simulink model "Centralized_Control_G18"  (R2020a)
settings: Solver=VariableStepAuto  StartTime=0.0  StopTime=60  RelTol=1e-3
values from neighbouring files (symbols this model uses):
  CK_dH = CK_dL.*5    [Dynamics_G18.m]
  CK_dL = diag([40; 40; 40; 40; 40; 40])    [Dynamics_G18.m]
  CK_dM = CK_dL.*3    [Dynamics_G18.m]
  CK_pH = CK_pL.*25    [Dynamics_G18.m]
  CK_pL = diag([400; 400; 400; 400; 400; 400])    [Dynamics_G18.m]
  CK_pM = CK_pL.*9    [Dynamics_G18.m]
  DH = [ 0.089    q1     0    pi/2    0     'R' ... (first row only)    [Robot_G18.m]
libraries: vrlib x7, dspinverses x2, aerolibanimutils x1, RobotG18_Blocos x1, simulink x1
settings Model: Creator=Ricardo Henriques  LastModifiedBy=Catarina
settings DataIOCC: ReturnWorkspaceOutputs=off
settings OptimizationCC: LifeSpan=inf
settings DebuggingCC: ArithmeticOperatorsInVariantConditions=warning
settings SFSimCC: SimUseLocalCustomCode=off  CustomCodeUndefinedFunction=UseInterfaceOnly
settings RTWCC: RTWUseLocalCustomCode=off
settings CodeAppCC: StateflowObjectComments=on

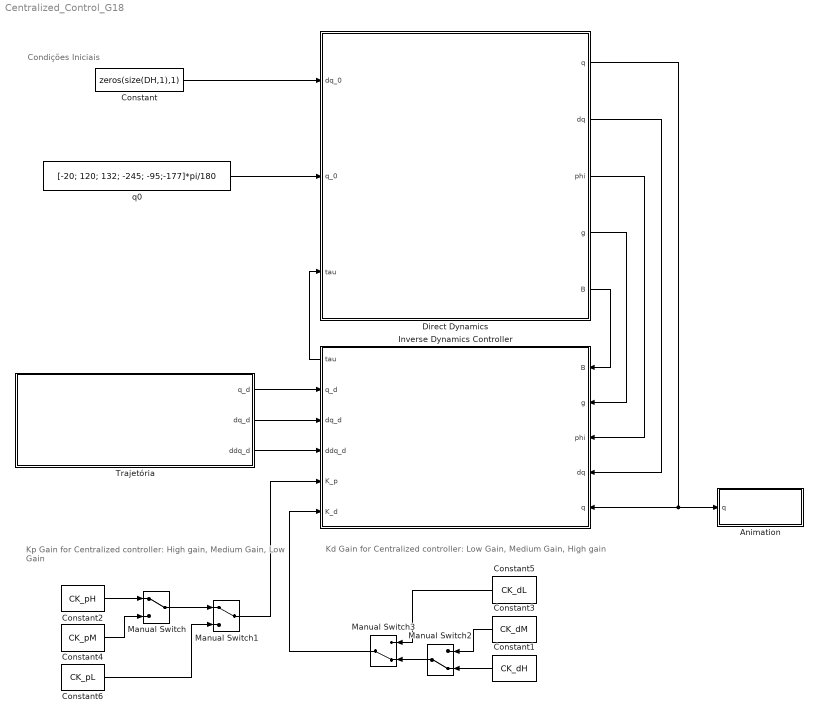
== system Centralized_Control_G18 ==
  note: Kd Gain for Centralized controller:
      |  Low Gain, Medium Gain, High gain
  note: Kp Gain for Centralized controller:
      | High gain, Medium Gain, Low Gain
  note: Condições Iniciais
  "Animation " : Subsystem
  Constant : Constant  Value=zeros(size(DH,1),1)  VectorParams1D=off
  Constant1 : Constant  Value=CK_dH  VectorParams1D=off
  Constant2 : Constant  Value=CK_pH  VectorParams1D=off
  Constant3 : Constant  Value=CK_dM  VectorParams1D=off
  Constant4 : Constant  Value=CK_pM  VectorParams1D=off
  Constant5 : Constant  Value=CK_dL  VectorParams1D=off
  Constant6 : Constant  Value=CK_pL  VectorParams1D=off
  Direct Dynamics : Subsystem
  Inverse Dynamics Controller : Subsystem
      settings: PortSchema="{\"entries\":[{\"content\":{\"sides\":[{\"content\":{\"connectorIds\":[\"In1\",\"In2\",\"In3\",\"In4\",\"In5\"]},\"type\":\"ConnectorPlacement.EquallySpacedRectSide\",\"uuid\":\"0e680a2d-49f3-406c-b827-b0951d4aa640\"},{\"content\":{\"connectorIds\":[\"Out1\",\"In6\",\"In7\",\"In8\",\"In9\",\"In10\"],\"side\":\"RIGHT\"},\"type\":\"ConnectorPlacement.EquallySpacedRectSide\",\"uuid\":\"bf9b0e73-475c-43b8-a2d1-242f88155fc5\"},{\"content\":{\"connectorIds\":[],\"side\":\"TOP\"},\"type\":\"ConnectorPlacement.EquallySpacedRectSide\",\"uuid\":\"dd2b5620-6d82-4ff2-af29-930996194164\"}]},\"type\":\"ConnectorPlacement.EquallySpacedConnector\",\"uuid\":\"c87e6944-d8f4-4feb-bccd-937ad879e06a\"}],\"packageUris\":[\"http://schema.mathworks.com/mf0/Connector/19700101\"],\"version\":\"1.0\"}"
  Manual Switch : ManualSwitch
  Manual Switch1 : ManualSwitch
  Manual Switch2 : ManualSwitch  CurrentSetting=0
  Manual Switch3 : ManualSwitch  CurrentSetting=0
  Trajetória : Subsystem
  q0 : Constant  Value=[-20; 120; 132; -245; -95;-177]*pi/180  VectorParams1D=off
  wires:
  Constant/1 -> Direct Dynamics/1(dq_0)
  Direct Dynamics/5(B) -> Inverse Dynamics Controller/1(B)
  Direct Dynamics/4(g) -> Inverse Dynamics Controller/2(g)
  Direct Dynamics/3(phi) -> Inverse Dynamics Controller/3(phi)
  Direct Dynamics/2(dq) -> Inverse Dynamics Controller/4(dq)
  Direct Dynamics/1(q) -> "Animation "/1("q "), Inverse Dynamics Controller/5(q)
  Inverse Dynamics Controller/1(tau) -> Direct Dynamics/3(tau)
  q0/1 -> Direct Dynamics/2(q_0)
  Trajetória/3(ddq_d) -> Inverse Dynamics Controller/8(ddq_d)
  Constant2/1 -> Manual Switch/1
  Constant4/1 -> Manual Switch/2
  Manual Switch/1 -> Manual Switch1/1
  Manual Switch1/1 -> Inverse Dynamics Controller/9(K_p)
  Constant6/1 -> Manual Switch1/2
  Constant1/1 -> Manual Switch2/2
  Constant3/1 -> Manual Switch2/1
  Manual Switch2/1 -> Manual Switch3/2
  Manual Switch3/1 -> Inverse Dynamics Controller/10(K_d)
  Constant5/1 -> Manual Switch3/1
  Trajetória/2(dq_d) -> Inverse Dynamics Controller/7(dq_d)
  Trajetória/1(q_d) -> Inverse Dynamics Controller/6(q_d)

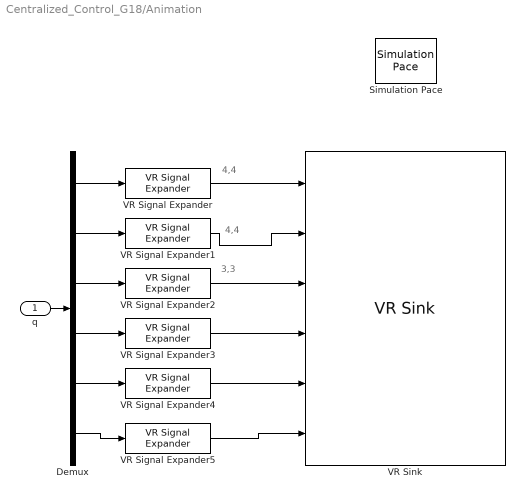
== system Centralized_Control_G18/Animation  ==
  note: 4,4
  note: 3,3
  note: 4,4
  "q " : Inport
  Demux : Demux  Outputs=6
  Simulation Pace : aerolibanimutils/Simulation Pace  SimulationPace=1  SleepMode=Auto  OutputPaceError=off  SampleTime=1/30
  VR Signal Expander{,1..5} (6 alike) : vrlib/VR Signal Expander  outwidth=4  outidx=4
  VR Sink : vrlib/VR Sink  InstantiateOnLoad=on  SampleTime=1/30  ViewEnable=on  RemoteChange=off  RemoteView=off  FieldsWritten=Jt1_DH_dv.rotation.4.1.1.double#Jt2_DH_dv.rotation.4.1.1.double#Jt3_DH_dv.rotation.4.1.1.double#Jt4_DH_dv.rotation.4.1.1.double#Jt5_DH_dv.rotation.4.1.1.double#Jt6_DH_dv.rotation.4.1.1.double  WorldFileName=RobotG18_Opt_NoAxes.wrl  WorldDescription=D-H Reference Frames for Virtual Reality Robot  AutoView=off  VideoDimensions=[]  AllowVariableSize=off
  wires:
  "q "/1 -> Demux/1
  Demux/1 -> VR Signal Expander/1
  Demux/2 -> VR Signal Expander1/1
  Demux/3 -> VR Signal Expander2/1
  Demux/4 -> VR Signal Expander3/1
  Demux/5 -> VR Signal Expander4/1
  Demux/6 -> VR Signal Expander5/1
  VR Signal Expander/1 -> VR Sink/1
  VR Signal Expander1/1 -> VR Sink/2
  VR Signal Expander5/1 -> VR Sink/6
  VR Signal Expander2/1 -> VR Sink/3
  VR Signal Expander3/1 -> VR Sink/4
  VR Signal Expander4/1 -> VR Sink/5

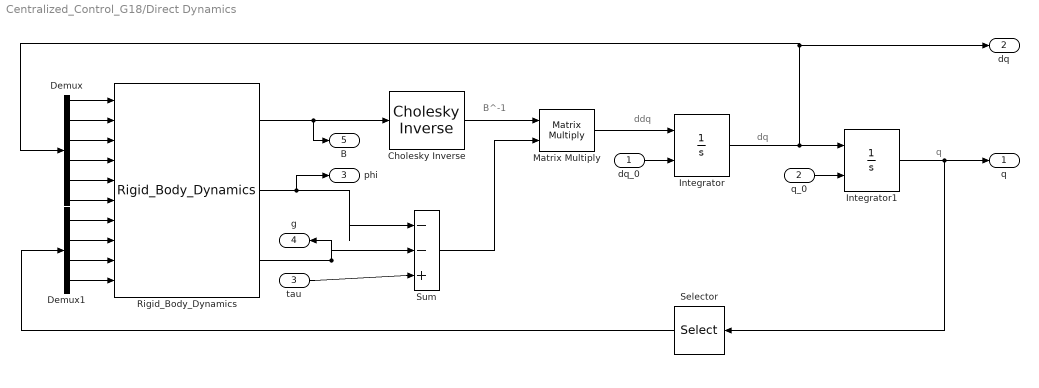
== system Centralized_Control_G18/Direct Dynamics ==
  note: q
  note: dq
  note: ddq
  note: B^-1
  dq_0 : Inport
  q_0 : Inport  Port=2
  tau : Inport  Port=3
  Cholesky Inverse : dspinverses/Cholesky Inverse  errmode=Warning
      settings: SourceProductBaseCode=DS
  Demux : Demux  Outputs=6
  Demux1 : Demux
  Integrator : Integrator  InitialConditionSource=external
  Integrator1 : Integrator  InitialConditionSource=external
  Matrix Multiply : Product  Multiplication=Matrix(*)
  Rigid_Body_Dynamics : RobotG18_Blocos/Rigid_Body_Dynamics  SystemSampleTime=-1  Latency=0  AutoFrameSizeCalculation=off
  Selector : Selector  InputPortWidth=6  IndexOptions=Index vector (dialog)  Indices=[2 3 4 5]  OutputSizes=1
  Sum : Sum  Inputs=|--+
  q : Outport
  dq : Outport  Port=2
  phi : Outport  Port=3
  g : Outport  Port=4
  B : Outport  Port=5
  wires:
  dq_0/1 -> Integrator/2
  Integrator1/1 -> q/1, Selector/1
  q_0/1 -> Integrator1/2
  Matrix Multiply/1 -> Integrator/1
  Cholesky Inverse/1 -> Matrix Multiply/1
  Sum/1 -> Matrix Multiply/2
  Rigid_Body_Dynamics/1 -> B/1, Cholesky Inverse/1
  tau/1 -> Sum/3
  Rigid_Body_Dynamics/3 -> g/1, Sum/2
  Rigid_Body_Dynamics/2 -> phi/1, Sum/1
  Demux/1 -> Rigid_Body_Dynamics/1
  Demux/2 -> Rigid_Body_Dynamics/2
  Demux/3 -> Rigid_Body_Dynamics/3
  Demux/4 -> Rigid_Body_Dynamics/4
  Demux/5 -> Rigid_Body_Dynamics/5
  Demux/6 -> Rigid_Body_Dynamics/6
  Demux1/1 -> Rigid_Body_Dynamics/7
  Demux1/2 -> Rigid_Body_Dynamics/8
  Demux1/3 -> Rigid_Body_Dynamics/9
  Demux1/4 -> Rigid_Body_Dynamics/10
  Selector/1 -> Demux1/1
  Integrator/1 -> Demux/1, dq/1, Integrator1/1

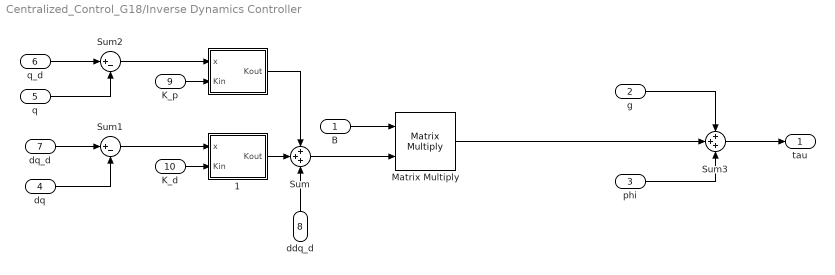
== system Centralized_Control_G18/Inverse Dynamics Controller ==
  B : Inport
  g : Inport  Port=2
  phi : Inport  Port=3
  dq : Inport  Port=4
  q : Inport  Port=5
  q_d : Inport  Port=6
  dq_d : Inport  Port=7
  ddq_d : Inport  Port=8
  K_p : Inport  Port=9
  K_d : Inport  Port=10
  " " : MATLAB Function  TreatAsAtomicUnit=on
  " 1" : MATLAB Function  TreatAsAtomicUnit=on
  Matrix Multiply : Product  Multiplication=Matrix(*)
  Sum : Sum  Inputs=+++
  Sum1 : Sum  Inputs=|+-
  Sum2 : Sum  Inputs=|+-
  Sum3 : Sum  Inputs=+++
  tau : Outport
  wires:
  Sum1/1 -> " 1"/1(x)
  Sum/1 -> Matrix Multiply/2
  ddq_d/1 -> Sum/3
  " 1"/1(Kout) -> Sum/2
  dq_d/1 -> Sum1/1
  Sum2/1 -> " "/1(x)
  q_d/1 -> Sum2/1
  Sum3/1 -> tau/1
  g/1 -> Sum3/1
  B/1 -> Matrix Multiply/1
  phi/1 -> Sum3/3
  Matrix Multiply/1 -> Sum3/2
  q/1 -> Sum2/2
  dq/1 -> Sum1/2
  " "/1(Kout) -> Sum/1
  K_p/1 -> " "/2(Kin)
  K_d/1 -> " 1"/2(Kin)

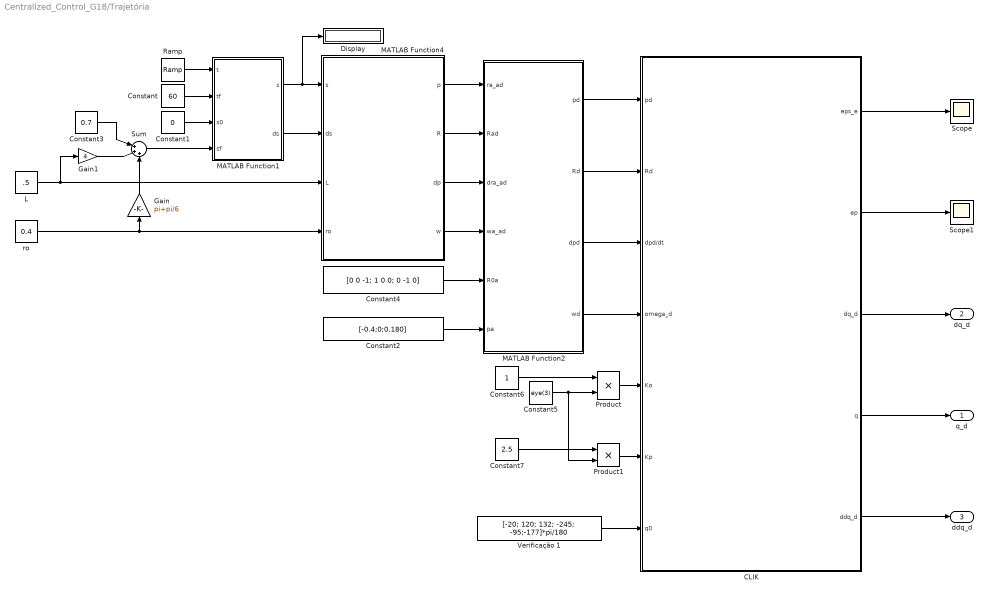
== system Centralized_Control_G18/Trajetória ==
  CLIK : Subsystem
  Constant : Constant  Value=60
  Constant1 : Constant  Value=0
  Constant2 : Constant  Value=[-0.4;0;0.180]  VectorParams1D=off
  Constant3 : Constant  Value=0.7
  Constant4 : Constant  Value=[0 0 -1; 1 0 0; 0 -1 0]  VectorParams1D=off
  Constant5 : Constant  Value=eye(3)
  Constant6 : Constant
  Constant7 : Constant  Value=2.5
  Display : Display
  Gain : Gain  Gain=pi+pi/6
  Gain1 : Gain  Gain=4
  L : Constant  Value=.5
  MATLAB Function1 : MATLAB Function  TreatAsAtomicUnit=on
  MATLAB Function2 : MATLAB Function  TreatAsAtomicUnit=on
  MATLAB Function4 : MATLAB Function  TreatAsAtomicUnit=on
  Product : Product
  Product1 : Product
  Ramp : simulink/Sources/Ramp  slope=1  start=0  InitialOutput=0
  Scope : Scope
  Scope1 : Scope
  Sum : Sum  Inputs=|+++
  Verificação 1 : Constant  Value=[-20; 120; 132; -245; -95;-177]*pi/180  VectorParams1D=off  SampleTime=inf
  ro : Constant  Value=0.4
  q_d : Outport
  dq_d : Outport  Port=2
  ddq_d : Outport  Port=3
  wires:
  MATLAB Function2/2(Rd) -> CLIK/2(Rd)
  Product1/1 -> CLIK/6(Kp)
  Constant4/1 -> MATLAB Function2/5(R0a)
  Gain/1 -> Sum/3
  CLIK/3(dq_d) -> dq_d/1
  CLIK/2(ep) -> Scope1/1
  CLIK/4(q) -> q_d/1
  Constant/1 -> MATLAB Function1/2(tf)
  Constant1/1 -> MATLAB Function1/3(s0)
  CLIK/1(eps_e) -> Scope/1
  Constant3/1 -> Sum/1
  Constant7/1 -> Product1/1
  MATLAB Function4/4(w) -> MATLAB Function2/4(wa_ad)
  Constant6/1 -> Product/1
  MATLAB Function1/2(ds) -> MATLAB Function4/2(ds)
  MATLAB Function2/3(dpd) -> CLIK/3(dpd/dt)
  Verificação 1/1 -> CLIK/7(q0)
  Sum/1 -> MATLAB Function1/4(sf)
  ro/1 -> MATLAB Function4/4(ro), Gain/1
  MATLAB Function4/3(dp) -> MATLAB Function2/3(dra_ad)
  MATLAB Function2/1(pd) -> CLIK/1(pd)
  Ramp/1 -> MATLAB Function1/1(t)
  Constant5/1 -> Product1/2, Product/2
  Constant2/1 -> MATLAB Function2/6(pa)
  MATLAB Function2/4(wd) -> CLIK/4(omega_d)
  Product/1 -> CLIK/5(Ko)
  MATLAB Function4/1(p) -> MATLAB Function2/1(ra_ad)
  Gain1/1 -> Sum/2
  MATLAB Function1/1(s) -> MATLAB Function4/1(s), Display/1
  MATLAB Function4/2(R) -> MATLAB Function2/2(Rad)
  L/1 -> MATLAB Function4/3(L), Gain1/1
  CLIK/5(ddq_d) -> ddq_d/1

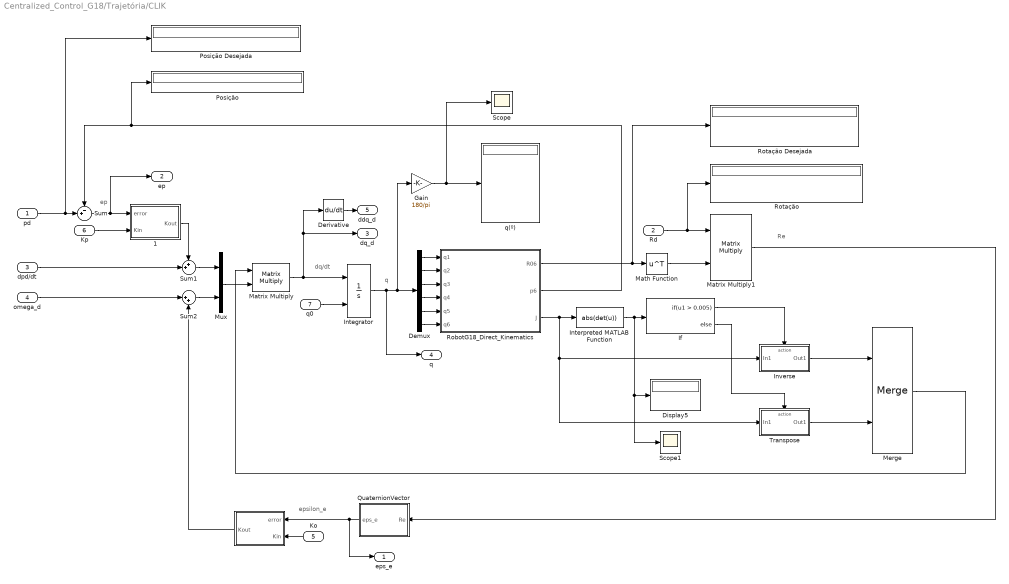
== system Centralized_Control_G18/Trajetória/CLIK ==
  note: epsilon_e
  note: Re
  note: ep
  note: dq/dt
  note: q
  pd : Inport
  Rd : Inport  Port=2
  dpd/dt : Inport  Port=3
  omega_d : Inport  Port=4
  Ko : Inport  Port=5
  Kp : Inport  Port=6
  q0 : Inport  Port=7
  " " : MATLAB Function  TreatAsAtomicUnit=on
  " 1" : MATLAB Function  TreatAsAtomicUnit=on
  Demux : Demux  Outputs=6
  Derivative : Derivative
  Display5 : Display
  Gain : Gain  Gain=180/pi
  If : If  IfExpression=u1 > 0.005  ZeroCross=off
  Integrator : Integrator  InitialConditionSource=external
  Interpreted MATLAB Function : MATLABFcn  MATLABFcn=abs(det(u))
  Inverse : Subsystem  TreatAsAtomicUnit=on
  Math Function : Math  Operator=transpose  SignedPower=on  SaturateOnIntegerOverflow=on
  Matrix Multiply : Product  Multiplication=Matrix(*)
  Matrix Multiply1 : Product  Multiplication=Matrix(*)
  Merge : Merge
  Mux : Mux  Inputs=2
  Posição : Display
      settings: Decimation=3
  Posição Desejada : Display
      settings: Decimation=3
  QuaternionVector : MATLAB Function  TreatAsAtomicUnit=on
  RobotG18_Direct_Kinematics : MATLAB Function  TreatAsAtomicUnit=on
  Rotação : Display
      settings: Decimation=3
  Rotação Desejada : Display
      settings: Decimation=3
  Scope : Scope
  Scope1 : Scope
  Sum : Sum  Inputs=-+|
  Sum1 : Sum  Inputs=++|
  Sum2 : Sum  Inputs=|++
  Transpose : Subsystem  TreatAsAtomicUnit=on
  q(º) : Display
  eps_e : Outport
  ep : Outport  Port=2
  dq_d : Outport  Port=3
  q : Outport  Port=4
  ddq_d : Outport  Port=5
  wires:
  Integrator/1 -> q/1, Gain/1, Demux/1
  Demux/3 -> RobotG18_Direct_Kinematics/3(q3)
  Demux/4 -> RobotG18_Direct_Kinematics/4(q4)
  Demux/1 -> RobotG18_Direct_Kinematics/1(q1)
  Demux/2 -> RobotG18_Direct_Kinematics/2(q2)
  Demux/5 -> RobotG18_Direct_Kinematics/5(q5)
  Demux/6 -> RobotG18_Direct_Kinematics/6(q6)
  QuaternionVector/1(eps_e) -> " "/1(error), eps_e/1
  Matrix Multiply/1 -> Derivative/1, dq_d/1, Integrator/1
  Math Function/1 -> Matrix Multiply1/2
  " "/1(Kout) -> Sum2/2
  omega_d/1 -> Sum2/1
  Sum2/1 -> Mux/2
  Sum1/1 -> Mux/1
  Mux/1 -> Matrix Multiply/2
  Rd/1 -> Rotação/1, Matrix Multiply1/1
  Matrix Multiply1/1 -> QuaternionVector/1(Re)
  pd/1 -> Posição Desejada/1, Sum/2
  RobotG18_Direct_Kinematics/2(p6) -> Posição/1, Sum/1
  Sum/1 -> " 1"/1(error), ep/1
  dpd/dt/1 -> Sum1/2
  RobotG18_Direct_Kinematics/1(R06) -> Math Function/1, Rotação Desejada/1
  RobotG18_Direct_Kinematics/3(J) -> Interpreted MATLAB Function/1, Inverse/1(In1), Transpose/1(In1)
  If/1 -> Inverse/Action
  If/2 -> Transpose/Action
  Transpose/1(Out1) -> Merge/2
  Inverse/1(Out1) -> Merge/1
  Merge/1 -> Matrix Multiply/1
  Gain/1 -> Scope/1, q(º)/1
  q0/1 -> Integrator/2
  Ko/1 -> " "/2(Kin)
  " 1"/1(Kout) -> Sum1/1
  Kp/1 -> " 1"/2(Kin)
  Interpreted MATLAB Function/1 -> Scope1/1, Display5/1, If/1
  Derivative/1 -> ddq_d/1

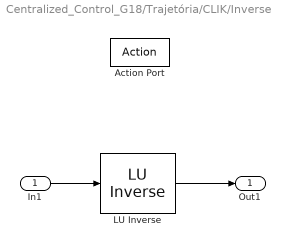
== system Centralized_Control_G18/Trajetória/CLIK/Inverse ==
  In1 : Inport
  Action Port : ActionPort  ActionPortLabel=if(u1 > 0.005)
  " LU Inverse" : dspinverses/ LU Inverse
  Out1 : Outport
  wires:
  In1/1 -> " LU Inverse"/1
  " LU Inverse"/1 -> Out1/1

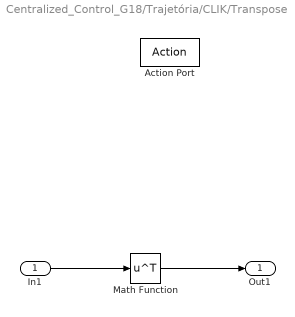
== system Centralized_Control_G18/Trajetória/CLIK/Transpose ==
  In1 : Inport
  Action Port : ActionPort  ActionPortLabel=else
  Math Function : Math  Operator=transpose  SignedPower=on  SaturateOnIntegerOverflow=on
  Out1 : Outport
  wires:
  In1/1 -> Math Function/1
  Math Function/1 -> Out1/1

== matlab function Centralized_Control_G18/Inverse Dynamics Controller/  ==
  data: x input; Kin input; Kout output
function Kout = Gains(x, Kin)

Kout = Kin*x;

== matlab function Centralized_Control_G18/Inverse Dynamics Controller/ 1 ==
  data: x input; Kin input; Kout output
function Kout = Gains(x, Kin)

Kout = Kin*x;

== matlab function Centralized_Control_G18/Trajetória/CLIK/  ==
  data: error input; Kin input; Kout output
function Kout = Gains(error, Kin)

Kout = Kin*error;

== matlab function Centralized_Control_G18/Trajetória/CLIK/ 1 ==
  data: error input; Kin input; Kout output
function Kout = Gains(error, Kin)

Kout = Kin*error;

== matlab function Centralized_Control_G18/Trajetória/CLIK/QuaternionVector ==
  data: Re input; eps_e output
function eps_e  = QuaternionVector(Re)

eps_e = 0.5 * [sign(Re(3,2)-Re(2,3)) * sqrt(abs(Re(1,1)-Re(2,2)-Re(3,3)+1));
               sign(Re(1,3)-Re(3,1)) * sqrt(abs(Re(2,2)-Re(1,1)-Re(3,3)+1));
               sign(Re(2,1)-Re(1,2)) * sqrt(abs(Re(3,3)-Re(1,1)-Re(2,2)+1))];
           
end

== matlab function Centralized_Control_G18/Trajetória/CLIK/RobotG18_Direct_Kinematics ==
  data: q1 input; R06 output; q2 input; q3 input; q4 input; q5 input; q6 input; p6 output; J output
function [R06,p6,J] = RobotG18_Direct_Kinematics(q1,q2,q3,q4,q5,q6)
%#codegen

%    This function was generated by the Symbolic Math Toolbox version 7.0.
%    15-Apr-2021 18:49:51

t2 = q2+q3+q4;
t3 = cos(q1);
t4 = sin(q6);
t5 = sin(q1);
t6 = sin(q5);
t7 = t5.*t6;
t8 = cos(t2);
t9 = cos(q5);
t10 = t7-t3.*t8.*t9;
t11 = sin(t2);
t12 = cos(q6);
t13 = t3.*t6;
t14 = t5.*t8.*t9;
t15 = t13+t14;
t16 = q2+q3;
t17 = cos(q2);
t18 = sin(q2);
t19 = sin(q3);
t20 = cos(t16);
t21 = sin(q4);
t22 = sin(t16);
t23 = cos(q4);
t24 = cos(q3);
t25 = t5.*t17.*(1.7e1./4.0e1);
t26 = t5.*t6.*t8.*(4.1e1./5.0e2);
t27 = t5.*t17.*t24.*(4.9e1./1.25e2);
t28 = t22.*(4.9e1./1.25e2);
t29 = t18.*(1.7e1./4.0e1);
t30 = t20.*t21.*(4.1e1./5.0e2);
t31 = t22.*t23.*(4.1e1./5.0e2);
t32 = t30+t31;
t33 = t6.*t32;
t34 = t20.*t23.*(1.9e1./2.0e2);
t35 = t8.*(1.9e1./2.0e2);
t36 = t6.*t11.*(4.1e1./5.0e2);
t37 = t5.*(1.09e2./1.0e3);
t38 = t3.*t17.*(1.7e1./4.0e1);
t39 = t5.*t9.*(4.1e1./5.0e2);
t40 = t3.*t6.*t8.*(4.1e1./5.0e2);
t41 = t3.*t17.*t24.*(4.9e1./1.25e2);
t42 = t37+t38+t39+t40+t41-t3.*t18.*t19.*(4.9e1./1.25e2)-t3.*t20.*t21.*(1.9e1./2.0e2)-t3.*t22.*t23.*(1.9e1./2.0e2);
t43 = t28+t29+t33+t34-t21.*t22.*(1.9e1./2.0e2);
t44 = t28+t35+t36;
t45 = t35+t36;
t46 = q2+q3+q4+q5;
t47 = sin(t46);
t48 = t47.*(4.1e1./1.0e3);
t49 = t20.*(4.9e1./1.25e2);
t50 = q2+q3+q4-q5;
t51 = sin(t50);
t52 = t5.*t9;
t53 = t3.*t6.*t8;
t54 = t52+t53;
t55 = t5.*t6.*t8;
t56 = t55-t3.*t9;
t57 = t6.*t11;
R06 = reshape([-t10.*t12-t3.*t4.*t11,t12.*t15-t4.*t5.*t11,t4.*t8+t9.*t11.*t12,t4.*t10-t3.*t11.*t12,-t4.*t15-t5.*t11.*t12,t8.*t12-t4.*t9.*t11,t54,t56,t57],[3,3]);
if nargout > 1
    p6 = [t42;t3.*(-1.09e2./1.0e3)+t25+t26+t27-t3.*t9.*(4.1e1./5.0e2)-t5.*t18.*t19.*(4.9e1./1.25e2)-t5.*t20.*t21.*(1.9e1./2.0e2)-t5.*t22.*t23.*(1.9e1./2.0e2);t28+t29+t33+t34-t21.*t22.*(1.9e1./2.0e2)+8.9e1./1.0e3];
end
if nargout > 2
    J = reshape([t3.*(1.09e2./1.0e3)-t25-t26-t27+t3.*t9.*(4.1e1./5.0e2)+t5.*t18.*t19.*(4.9e1./1.25e2)+t5.*t20.*t21.*(1.9e1./2.0e2)+t5.*t22.*t23.*(1.9e1./2.0e2),t42,0.0,0.0,0.0,1.0,-t3.*t43,-t5.*t43,t11.*(-1.9e1./2.0e2)+t17.*(1.7e1./4.0e1)+t48+t49-t51.*(4.1e1./1.0e3),t5,-t3,0.0,-t3.*t44,-t5.*t44,t11.*(-1.9e1./2.0e2)+t48+t49-t51.*(4.1e1./1.0e3),t5,-t3,0.0,-t3.*t45,-t5.*t45,t11.*(-1.9e1./2.0e2)+t48-t51.*(4.1e1./1.0e3),t5,-t3,0.0,t5.*t6.*(-4.1e1./5.0e2)-t3.*t9.*t17.*t19.*t21.*(4.1e1./5.0e2)-t3.*t9.*t18.*t19.*t23.*(4.1e1./5.0e2)-t3.*t9.*t18.*t21.*t24.*(4.1e1./5.0e2)+t3.*t9.*t17.*t23.*t24.*(4.1e1./5.0e2),t3.*t6.*(4.1e1./5.0e2)-t5.*t9.*t17.*t19.*t21.*(4.1e1./5.0e2)-t5.*t9.*t18.*t19.*t23.*(4.1e1./5.0e2)-t5.*t9.*t18.*t21.*t24.*(4.1e1./5.0e2)+t5.*t9.*t17.*t23.*t24.*(4.1e1./5.0e2),t48+t51.*(4.1e1./1.0e3),-t3.*t11,-t5.*t11,t8,0.0,0.0,0.0,t54,t56,t57],[6,6]);
end

== matlab function Centralized_Control_G18/Trajetória/MATLAB Function1 ==
  data: t input; s output; tf input; s0 input; sf input; ds output
function [s,ds] = length(t,tf,s0,sf)
if t<=tf
    s=s0+3*(sf-s0)*(t/tf)^2-2*(sf-s0)*(t/tf)^3;
    
    ds = 6*(sf-s0)*t/tf^2-6*(sf-s0)*t^2/tf^3;
else
    s=sf;
    ds=0;
end
end

== matlab function Centralized_Control_G18/Trajetória/MATLAB Function2 ==
  data: ra_ad input; pd output; Rad input; dra_ad input; wa_ad input; R0a input; pa input; Rd output; dpd output; wd output
function [pd,Rd,dpd,wd]=fcn(ra_ad,Rad,dra_ad,wa_ad,R0a,pa)

pd = pa+R0a*ra_ad;
Rd = R0a*Rad;
dpd = R0a*dra_ad;
wd = R0a*wa_ad;

== matlab function Centralized_Control_G18/Trajetória/MATLAB Function4 ==
  data: p output; R output; s input; ds input; L input; ro input; dp output; w output
function [p,R,dp,w] = trajectory(s,ds,L,ro)

p=zeros(3,1);
R=eye(3);
dp=zeros(3,1);
w=zeros(3,1);

if 0 <= s && s<= L
%% Path 1 ------- Subida ---------
    p=[0;-s;0];
    R=[1 0 0; 0 1 0; 0 0 1];
    
    dp=[0;-ds;0];
    w=zeros(3,1);
    
elseif L < s && s <= L+((pi/2)*ro)
%% Path 2  ------- Roda ---------
    p=[ro*sin((s-L)/ro);
        -L;
        -ro+ro*cos((s-L)/ro)];
    
    R=[ cos((s-L)/ro)   0   sin((s-L)/ro);
             0          1          0
       -sin((s-L)/ro)   0   cos((s-L)/ro)];
    
    dp = ds*[cos((s-L)/ro);0;-sin((s-L)/ro)];
    
    dR = (ds/ro)*[-sin((s-L)/ro)  0  cos((s-L)/ro);
                       0          1       0
                  -cos((s-L)/ro)   0  -sin((s-L)/ro)];
    Sw=dR*R';
    
    w = [Sw(3,2);Sw(1,3);Sw(2,1)];
    
elseif L+((pi/2)*ro) < s && s <= (2*L+((pi/2)*ro))
%% Path 3  ------- Descida ---------
    p = [ro;s-((2*L)+((pi/2)*ro));-ro];
    R = [0 0 1; 0 1 0; -1 0 0];
    
    dp = [0;ds;0];
    w = zeros(3,1);
    
elseif (2*L+((pi/2)*ro)) < s && s <= (2*L+((pi/2)*ro))+0.2
%% Path 4   ------- Estica (Coloca produto) ---------
    p = [(s-((2*L)+((pi/2)*ro)))+ro;0;-ro];
    R = [0 0 1; 0 1 0; -1 0 0];
    
    dp = [ds;0;0];
    w = zeros(3,1);
    
elseif (2*L+((pi/2)*ro))+0.2 < s && s <= (2*L+((pi/2)*ro))+0.5
%% Path 5  ------- Tempo de espera (larga produto) ---------
    p = [ro+0.2;0;-ro];
    R = [0 0 1; 0 1 0; -1 0 0];
    
    dp = [0;0;0];
    w = zeros(3,1);
    
elseif (2*L+((pi/2)*ro))+0.5 < s && s <= (2*L+((pi/2)*ro)+0.7)
%% Path 6   ------- Recolhe ---------
    p = [-(s-((2*L)+((pi/2)*ro)+0.7))+ro;0;-ro];
    R = [0 0 1; 0 1 0; -1 0 0];
    
    dp = [-ds;0;0];
    w = zeros(3,1);
    
elseif (2*L+((pi/2)*ro)+0.7) < s && s <= (3*L+((pi/2)*ro)+0.7)
    %% Path 7   ------- Subida ---------
    p = [ro;-(s-(2*L+((pi/2)*ro)+0.7));-ro];
    R = [0 0 1; 0 1 0; -1 0 0];
    
    dp = [0;-ds;0];
    w = zeros(3,1);
    

elseif (3*L+((pi/2)*ro)+0.7) < s && s <= (3*L+2*((pi/2)*ro)+0.7)
%% Path 8      ------- Roda de volta ---------
    p=[ro*sin((s-3*L-0.7)/ro);
        -L;
        -ro-ro*cos((s-3*L-0.7)/ro)];
    
    R=[ -cos((s-3*L-0.7)/ro)   0   sin((s-3*L-0.7)/ro);
                 0          1          0
        -sin((s-3*L-0.7)/ro)   0    -cos((s-3*L-0.7)/ro)];
    
    dp = ds*[cos((s-3*L-0.7)/ro);0;sin((s-3*L-0.7)/ro)];
    
    dR = (ds/ro)*[sin((s-3*L-0.7)/ro)  0  cos((s-3*L-0.7)/ro);
                           0          1          0
                   -cos((s-3*L-0.7)/ro)  0  sin((s-3*L-0.7)/ro)];
    Sw=dR*R';
    
    w = [Sw(3,2);Sw(1,3);Sw(2,1)];
    

elseif (3*L+2*((pi/2)*ro)+0.7) < s && s <= (4*L+2*((pi/2)*ro)+0.7)
%% Path 9  ------- Descida ---------
    p=[0;s-(4*L+2*((pi/2)*ro)+0.7);0];
    R=[1 0 0; 0 1 0; 0 0 1];
    
    dp=[0;ds;0];
    w=zeros(3,1);
    
end
end
